simulink model "CustomSourceBlocks"  (Simulink 5.0)
settings: Solver=ode45  StartTime=0.0  StopTime=10.0  RelTol=1e-3
undefined symbols (not defined in the file or in its folder): Bm, c, Jm, k, Kamp, Kb, Km, La, M, r, Ra
libraries: simulink x1
settings Model: LastModifiedBy=bbschube  SaveTime=off  SaveOutput=off

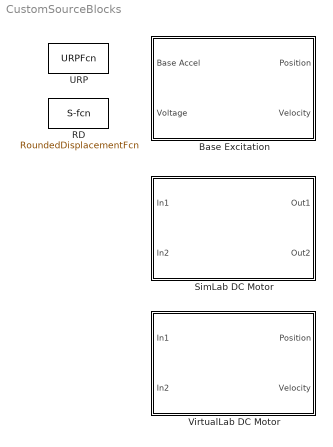
== system CustomSourceBlocks ==
  Base Excitation : Subsystem
  RD : S-Function  FunctionName=RoundedDisplacementFcn  Parameters=X, gw, Output, SampleTime  mask(Rounded Displacement (RD)){X=1, gw=5, Output=Acceleration, SampleTime=0}
      mask prompts: X "Amplitude:"; gw "Gamma*Omega:"; Output "Block Output:"; SampleTime "Sample Time"
      mask help: Output either the position, velocity or acceleration of the Rounded Displacement function.
      mask init:
      | t = [0:0.01:1];
      | y = 1-(1+t.*8).*exp(-t.*8);
      mask Help:
      | Generate RD(t), RD'(t), or RD''(t).
      | 
      | 
      | Description:
      | RD(t) = A*(1-(1+gwt)e^(-gwt)), where A is the amplitude, g (gamma) is the intensity factor, w (omega) is the circular frequency.
      | 
      | 
      | Amplitude:
      | The amplitude of the pulse, a real number.
      | 
      | gw:
      | The intensity factor multiplied by the frequency (gamma*omega), where T = (2*pi)/gw.
      | 
      | Output:
      | Select whether to output the RD, or its first or second derivative (ie. position, velocity, or acceleration).
      mask StyleString: edit,edit,popup(Position|Velocity|Acceleration),edit
      mask Display: plot(t,y)
  SimLab DC Motor : Subsystem
      mask Display:
      | port_label('input', 1, 'Base Accel')
      | port_label('input', 2, 'Voltage')
      | port_label('output', 1, 'Position')
      | port_label('output', 2, 'Speed')
  URP : S-Function  FunctionName=URPFcn  Parameters=X, gw, Output, SampleTime  mask(Unidirectional Rounded Pulse (URP)){X=1, gw=5, Output=Position, SampleTime=0}
      mask prompts: X "Amplitude:"; gw "Gamma*Omega:"; Output "Block Output:"; SampleTime "Sample Time"
      mask help: Output either the position, velocity or acceleration of the Unidirectional Rounded Pulse function.
      mask init:
      | t = [0:0.01:1];
      | y = exp(2)/4*(11)^2*exp(-t.*11).*t.^2;
      mask Help:
      | Generate URP(t), URP'(t), or URP''(t).
      | 
      | 
      | Description:
      | URP(t) = A*(e^2)/4*(g*w*t)^2*e^-g*w*t, where A is the amplitude, g (gamma) is the intensity factor, w (omega) is the circular frequency.
      | 
      | 
      | Amplitude:
      | The amplitude of the pulse, a real number.
      | 
      | gw:
      | The intensity factor multiplied by the frequency (gamma*omega), where T = (2*pi)/gw.
      | 
      | Output:
      | Select whether to output the URP, or its first or second derivative (ie. position, velocity, or acceleration).
      mask StyleString: edit,edit,popup(Position|Velocity|Acceleration),edit
      mask Display: plot(t,y)
  VirtualLab DC Motor : Subsystem
      mask Display:
      | port_label('input', 1, 'Base Accel')
      | port_label('input', 2, 'Voltage')
      | port_label('output', 1, 'Position')
      | port_label('output', 2, 'Speed')

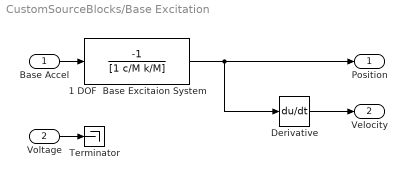
== system CustomSourceBlocks/Base Excitation ==
  Base Accel : Inport
  Voltage : Inport  Port=2
  1 DOF  Base Excitaion System : TransferFcn  Numerator=[-1]  Denominator=[1 c/M k/M]
  Derivative : Derivative
  Terminator : Terminator
  Position : Outport
  Velocity : Outport  Port=2
  wires:
  1 DOF  Base Excitaion System/1 -> Derivative/1, Position/1
  Derivative/1 -> Velocity/1
  Base Accel/1 -> 1 DOF  Base Excitaion System/1
  Voltage/1 -> Terminator/1

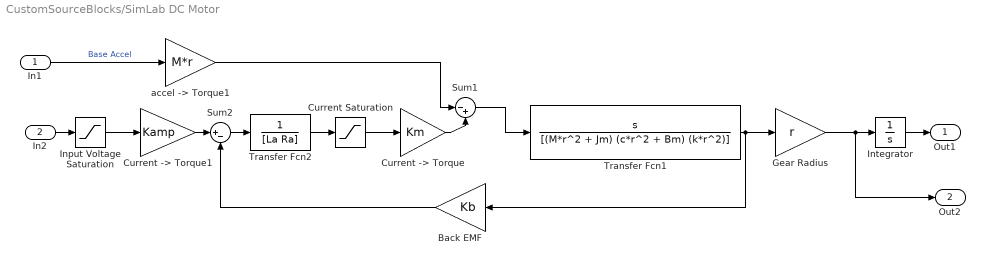
== system CustomSourceBlocks/SimLab DC Motor ==
  In1 : Inport
  In2 : Inport  Port=2
  Back EMF : Gain  Orientation=left  Gain=Kb  SaturateOnIntegerOverflow=on
  Current Saturation : Saturate  UpperLimit=+4  LowerLimit=-4
  "Current -> Torque" : Gain  Gain=Km  SaturateOnIntegerOverflow=on
  "Current -> Torque1" : Gain  Gain=Kamp  SaturateOnIntegerOverflow=on
  Gear Radius : Gain  Gain=r  SaturateOnIntegerOverflow=on
  Input Voltage Saturation : Saturate  UpperLimit=+10  LowerLimit=-10
  Integrator : Integrator
  Sum1 : Sum  Inputs=|-+  SaturateOnIntegerOverflow=on
  Sum2 : Sum  Inputs=|+-  SaturateOnIntegerOverflow=on
  Transfer Fcn1 : TransferFcn  Numerator=[1 0]  Denominator=[(M*r^2 + Jm) (c*r^2 + Bm) (k*r^2)]
  Transfer Fcn2 : TransferFcn  Denominator=[La Ra]
  "accel -> Torque1" : Gain  Gain=M*r  SaturateOnIntegerOverflow=on
  Out1 : Outport
  Out2 : Outport  Port=2
  wires:
  "Current -> Torque"/1 -> Sum1/2
  Input Voltage Saturation/1 -> "Current -> Torque1"/1
  Current Saturation/1 -> "Current -> Torque"/1
  "Current -> Torque1"/1 -> Sum2/1
  Back EMF/1 -> Sum2/2
  Sum2/1 -> Transfer Fcn2/1
  Transfer Fcn2/1 -> Current Saturation/1
  In1/1 -> "accel -> Torque1"/1  "Base Accel"
  In2/1 -> Input Voltage Saturation/1
  Transfer Fcn1/1 -> Back EMF/1, Gear Radius/1
  Sum1/1 -> Transfer Fcn1/1
  Integrator/1 -> Out1/1
  Gear Radius/1 -> Integrator/1, Out2/1
  "accel -> Torque1"/1 -> Sum1/1

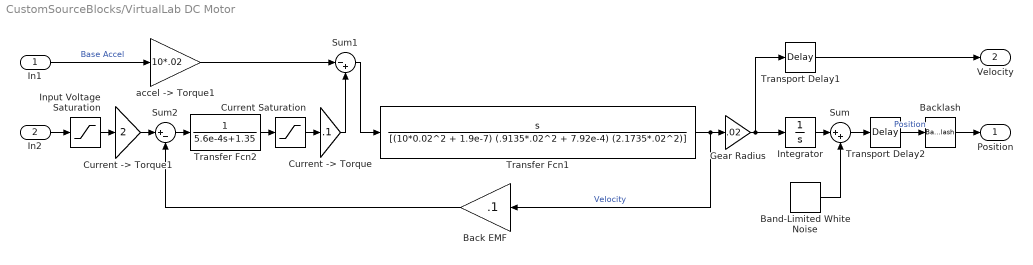
== system CustomSourceBlocks/VirtualLab DC Motor ==
  In1 : Inport
  In2 : Inport  Port=2
  Back EMF : Gain  Orientation=left  Gain=.1  SaturateOnIntegerOverflow=on
  Backlash : Backlash  BacklashWidth=0.0001
  Band-Limited White Noise : simulink/Sources/Band-Limited White Noise  Cov=0  Ts=0.01  seed=[23341]
  Current Saturation : Saturate  UpperLimit=+4  LowerLimit=-4
  "Current -> Torque" : Gain  Gain=.1  SaturateOnIntegerOverflow=on
  "Current -> Torque1" : Gain  Gain=2  SaturateOnIntegerOverflow=on
  Gear Radius : Gain  Gain=.02  SaturateOnIntegerOverflow=on
  Input Voltage Saturation : Saturate  UpperLimit=+10  LowerLimit=-10
  Integrator : Integrator
  Sum : Sum  Inputs=|++  SaturateOnIntegerOverflow=on
  Sum1 : Sum  Inputs=|-+  SaturateOnIntegerOverflow=on
  Sum2 : Sum  Inputs=|+-  SaturateOnIntegerOverflow=on
  Transfer Fcn1 : TransferFcn  Numerator=[1 0]  Denominator=[(10*0.02^2 + 1.9e-7) (.9135*.02^2 + 7.92e-4) (2.1735*.02^2)]
  Transfer Fcn2 : TransferFcn  Denominator=[5.6e-4 1.35]
  Transport Delay1 : TransportDelay  DelayTime=.001  BufferSize=4096
  Transport Delay2 : TransportDelay  DelayTime=.001  BufferSize=4096
  "accel -> Torque1" : Gain  Gain=10*.02  SaturateOnIntegerOverflow=on
  Position : Outport
  Velocity : Outport  Port=2
  wires:
  Transfer Fcn1/1 -> Back EMF/1, Gear Radius/1  "Velocity"
  Integrator/1 -> Sum/1
  Band-Limited White Noise/1 -> Sum/2
  Sum/1 -> Transport Delay2/1
  Transport Delay2/1 -> Backlash/1  "Position"
  "Current -> Torque"/1 -> Sum1/2
  Input Voltage Saturation/1 -> "Current -> Torque1"/1
  Current Saturation/1 -> "Current -> Torque"/1
  "Current -> Torque1"/1 -> Sum2/1
  Back EMF/1 -> Sum2/2
  Sum2/1 -> Transfer Fcn2/1
  Transfer Fcn2/1 -> Current Saturation/1
  In1/1 -> "accel -> Torque1"/1  "Base Accel"
  In2/1 -> Input Voltage Saturation/1
  Sum1/1 -> Transfer Fcn1/1
  Transport Delay1/1 -> Velocity/1
  Backlash/1 -> Position/1
  Gear Radius/1 -> Integrator/1, Transport Delay1/1
  "accel -> Torque1"/1 -> Sum1/1
